simulink model "idblocks"  (Simulink 6.3)
settings: Solver=ode45  StartTime=0.0  StopTime=10.0  RelTol=1e-3
values from neighbouring files (symbols this model uses):
  f = fn(1)    [fgnewt.m]    (also in m_mvid.m = TR*f*inv(TR))
  N = ss(AN,BN,CN,DN)    [ncf.m]
  q = TR*q    [m_mvid.m]
  Q = Q0*It; end    [adils.m]    (also in cfesens.m = [q1 q6;q2 q4;q3 q5]; dia_con.m = diag(x(1:m)); dia_con1.m = diag(x(1:m)); dia_conl.m = eye(m,m))
undefined symbols (not defined in the file or in its folder): f_ord, lambda, npar, QKF, rho, Tsa, u_noise, y_noise
libraries: simulink x22
settings Model: LastModifiedBy=Kostas Tsakalis  StrictBusMsg=None
settings OptimizationCC: InlineInvariantSignals=on

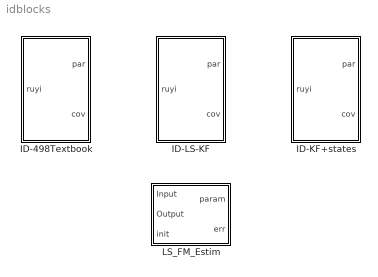
== system idblocks ==
  ID-498Textbook : Subsystem
  ID-KF+states : Subsystem
  ID-LS-KF : Subsystem
  LS_FM_Estim : Subsystem  mask{Tsa=0.01, N=4, thmin=-100, thmax=100, lambda=.9995, rho=1e5, y_noise=1e-6, u_noise=1e-6, Q=1e-8, lsgrad=1}
      mask prompts: Tsa "Tsample"; N "Order"; thmin "Min parameter"; thmax "Max Parameter"; rho "rho - Init cov"; y_noise "output regularization noise"; u_noise "input regularization noise"; Q "Q-dirft"; lsgrad "LS-gradient switch"

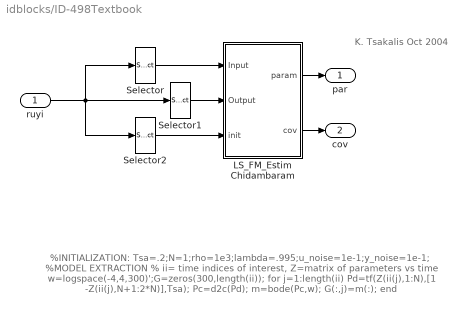
== system idblocks/ID-498Textbook ==
  note: %INITIALIZATION:
      | Tsa=.2;N=1;rho=1e3;lambda=.995;u_noise=1e-1;y_noise=1e-1;
      |
      | %MODEL EXTRACTION
      | % ii= time indices of interest, Z=matrix of parameters vs time
      | w=logspace(-4,4,300)';G=zeros(300,length(ii));
      | for j=1:length(ii)
      |    Pd=tf(Z(ii(j),1:N),[1 -Z(ii(j),N+1:2*N)],Tsa);
      |    Pc=d2c(Pd); m=bode(Pc,w); G(:,j)=m(:);
      | end
  note: K. Tsakalis
      | Oct 2004
  ruyi : Inport
  LS_FM_Estim Chidambaram : Subsystem
  Selector : Selector  Elements=2  InputPortWidth=4
  Selector1 : Selector  Elements=3  InputPortWidth=4
  Selector2 : Selector  Elements=4  InputPortWidth=4
  par : Outport
  cov : Outport  Port=2
  wires:
  Selector2/1 -> LS_FM_Estim Chidambaram/3(init)
  Selector1/1 -> LS_FM_Estim Chidambaram/2(Output)
  ruyi/1 -> Selector2/1, Selector1/1, Selector/1
  Selector/1 -> LS_FM_Estim Chidambaram/1(Input)
  LS_FM_Estim Chidambaram/1(param) -> par/1
  LS_FM_Estim Chidambaram/2(cov) -> cov/1

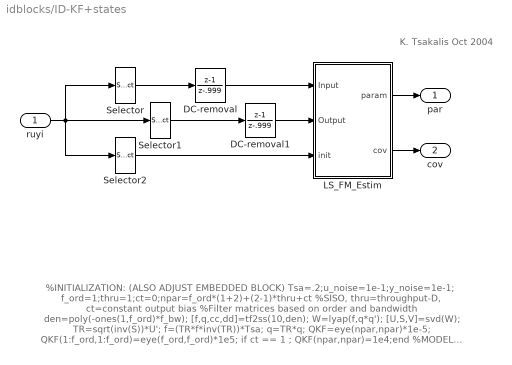
== system idblocks/ID-KF+states ==
  note: %INITIALIZATION: (ALSO ADJUST EMBEDDED BLOCK)
      | Tsa=.2;u_noise=1e-1;y_noise=1e-1;
      | f_ord=1;thru=1;ct=0;npar=f_ord*(1+2)+(2-1)*thru+ct
      | %SISO, thru=throughput-D, ct=constant output bias
      | %Filter matrices based on order and bandwidth
      | den=poly(-ones(1,f_ord)*f_bw); [f,q,cc,dd]=tf2ss(10,den);  W=lyap(f,q*q'); [U,S,V]=svd(W);
      | TR=sqrt(inv(S))*U';  f=(TR*f*inv(TR))*Tsa;  q=TR*q;
      | QKF=eye(npar,npar)*1e-5;   QKF(1:f_ord,1:f_ord)=eye(f_ord,f_ord)*1e5;
      | if ct == 1 ; QKF(npar,npar)=1e4;end
      |
      | %MODEL EXTRACTION
      | % ii= indices of points, Z=matrix of parameters vs time
      | w=logspace(-4,4,300)';G=zeros(300,length(ii));
      | for j=1:length(ii)
      |    q1=Z(ii(j),1:f_ord); q2=Z(ii(j),f_ord+1:2*f_ord); q3=Z(ii(j),mm-1*ct)*thru;
      |    Pd=ss(eye(size(f))+f'+q1'*q,q2'+q1'*q3,q,q3,Tsa); Pc=d2c(Pd); m=bode(Pc,w); G(:,j)=m(:);
      | end
  note: K. Tsakalis
      | Oct 2004
  ruyi : Inport
  DC-removal : DiscreteTransferFcn  Numerator=[1 -1]  Denominator=[1 -.999]  SampleTime=Tsa
  DC-removal1 : DiscreteTransferFcn  Numerator=[1 -1]  Denominator=[1 -.999]  SampleTime=Tsa
  LS_FM_Estim : Subsystem
  Selector : Selector  Elements=2  InputPortWidth=4
  Selector1 : Selector  Elements=3  InputPortWidth=4
  Selector2 : Selector  Elements=4  InputPortWidth=4
  par : Outport
  cov : Outport  Port=2
  wires:
  Selector2/1 -> LS_FM_Estim/3(init)
  Selector1/1 -> DC-removal1/1
  ruyi/1 -> Selector2/1, Selector1/1, Selector/1
  Selector/1 -> DC-removal/1
  LS_FM_Estim/1(param) -> par/1
  LS_FM_Estim/2(cov) -> cov/1
  DC-removal/1 -> LS_FM_Estim/1(Input)
  DC-removal1/1 -> LS_FM_Estim/2(Output)

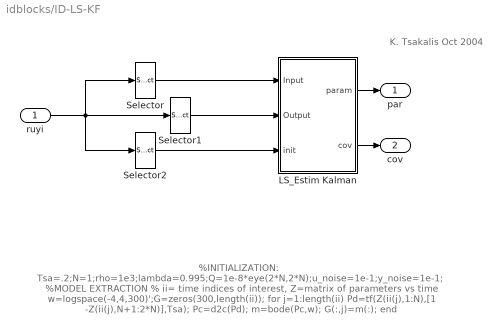
== system idblocks/ID-LS-KF ==
  note: %INITIALIZATION:
      | Tsa=.2;N=1;rho=1e3;lambda=0.995;Q=1e-8*eye(2*N,2*N);u_noise=1e-1;y_noise=1e-1;
      |
      | %MODEL EXTRACTION
      | % ii= time indices of interest, Z=matrix of parameters vs time
      | w=logspace(-4,4,300)';G=zeros(300,length(ii));
      | for j=1:length(ii)
      |    Pd=tf(Z(ii(j),1:N),[1 -Z(ii(j),N+1:2*N)],Tsa);
      |    Pc=d2c(Pd); m=bode(Pc,w); G(:,j)=m(:);
      | end
  note: K. Tsakalis
      | Oct 2004
  ruyi : Inport
  LS_Estim Kalman : Subsystem
  Selector : Selector  Elements=2  InputPortWidth=4
  Selector1 : Selector  Elements=3  InputPortWidth=4
  Selector2 : Selector  Elements=4  InputPortWidth=4
  par : Outport
  cov : Outport  Port=2
  wires:
  LS_Estim Kalman/2(cov) -> cov/1
  LS_Estim Kalman/1(param) -> par/1
  Selector/1 -> LS_Estim Kalman/1(Input)
  ruyi/1 -> Selector/1, Selector1/1, Selector2/1
  Selector1/1 -> LS_Estim Kalman/2(Output)
  Selector2/1 -> LS_Estim Kalman/3(init)

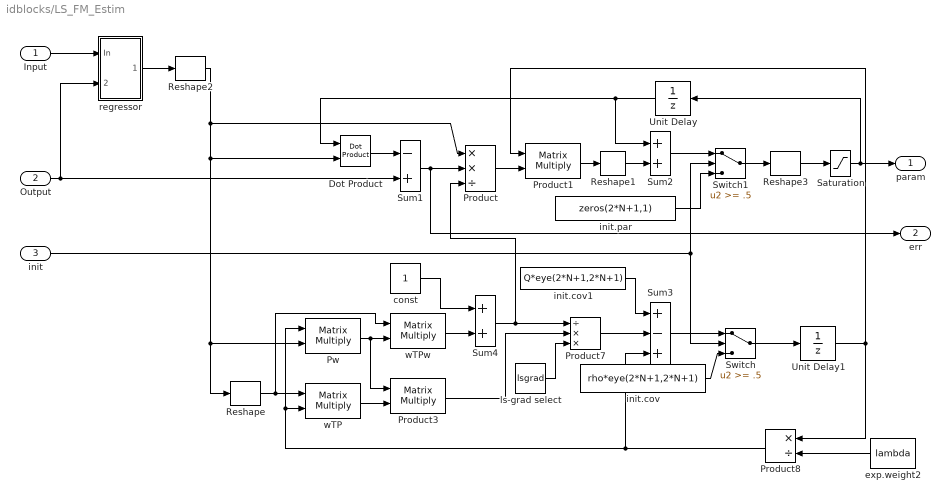
== system idblocks/LS_FM_Estim ==
  Input : Inport
  Output : Inport  Port=2
  init : Inport  Port=3
  Dot Product : simulink/Math Operations/Dot Product  InputSameDT=on  OutDataType=sfix(16)  OutScaling=2^-10  DoSatur=off
  Product : Product  Inputs=**/  RndMeth=Zero
  Product1 : Product  Multiplication=Matrix(*)  RndMeth=Zero
  Product3 : Product  Multiplication=Matrix(*)  RndMeth=Zero
  Product7 : Product  Inputs=/**  RndMeth=Zero
  Product8 : Product  Orientation=left  Inputs=*/  RndMeth=Zero
  Pw : Product  Multiplication=Matrix(*)  RndMeth=Zero
  Reshape : simulink/Math Operations/Reshape  OutputDimensionality=Row vector  OutputDimensions=[1,1]
  Reshape1 : simulink/Math Operations/Reshape  OutputDimensionality=Column vector  OutputDimensions=[1,1]
  Reshape2 : simulink/Math Operations/Reshape  OutputDimensionality=Column vector  OutputDimensions=[1,1]
  Reshape3 : simulink/Math Operations/Reshape  OutputDimensionality=1-D array  OutputDimensions=[1,1]
  Saturation : Saturate  UpperLimit=thmax  LowerLimit=thmin
  Sum1 : Sum  Inputs=-+  SaturateOnIntegerOverflow=on
  Sum2 : Sum  Inputs=2  SaturateOnIntegerOverflow=on
  Sum3 : Sum  Inputs=+-+  SaturateOnIntegerOverflow=on
  Sum4 : Sum  Inputs=2  SaturateOnIntegerOverflow=on
  Switch : Switch  Threshold=.5
  Switch1 : Switch  Threshold=.5
  Unit Delay : UnitDelay  Orientation=left  SampleTime=Tsa
  Unit Delay1 : UnitDelay  X0=rho*eye(2*N+1,2*N+1)  SampleTime=Tsa
  const : Constant
  exp.weight2 : Constant  Orientation=left  Value=lambda
  init.cov : Constant  Value=rho*eye(2*N+1,2*N+1)  VectorParams1D=off
  init.cov1 : Constant  Value=Q*eye(2*N+1,2*N+1)  VectorParams1D=off  SampleTime=Tsa
  init.par : Constant  Value=zeros(2*N+1,1)  VectorParams1D=off  SampleTime=Tsa
  ls-grad select : Constant  Value=lsgrad
  regressor : Subsystem
  wTP : Product  Multiplication=Matrix(*)  RndMeth=Zero
  wTPw : Product  Multiplication=Matrix(*)  RndMeth=Zero
  param : Outport
  err : Outport  Port=2
  wires:
  Saturation/1 -> Unit Delay/1, param/1
  Switch1/1 -> Reshape3/1
  init.cov1/1 -> Sum3/1
  Product7/1 -> Sum3/2
  exp.weight2/1 -> Product8/2
  Product8/1 -> Sum3/3, wTP/2, Pw/1
  ls-grad select/1 -> Product7/3
  Sum3/1 -> Switch/1
  const/1 -> Sum4/1
  regressor/1(regr) -> Reshape2/1
  Input/1 -> regressor/1(In)
  Reshape3/1 -> Saturation/1
  Reshape1/1 -> Sum2/2
  Dot Product/1 -> Sum1/1
  Output/1 -> regressor/2(out), Sum1/2
  Sum1/1 -> err/1, Product/2
  Product/1 -> Product1/2
  Reshape2/1 -> Dot Product/2, Reshape/1, Pw/2, Product/1
  Reshape/1 -> wTP/1, wTPw/1
  Product1/1 -> Reshape1/1
  wTP/1 -> Product3/2
  Product3/1 -> Product7/2
  Pw/1 -> Product3/1, wTPw/2
  wTPw/1 -> Sum4/2
  Sum4/1 -> Product/3, Product7/1
  Unit Delay1/1 -> Product8/1, Product1/1
  init.cov/1 -> Switch/3
  init/1 -> Switch/2, Switch1/2
  Switch/1 -> Unit Delay1/1
  Sum2/1 -> Switch1/1
  init.par/1 -> Switch1/3
  Unit Delay/1 -> Dot Product/1, Sum2/1

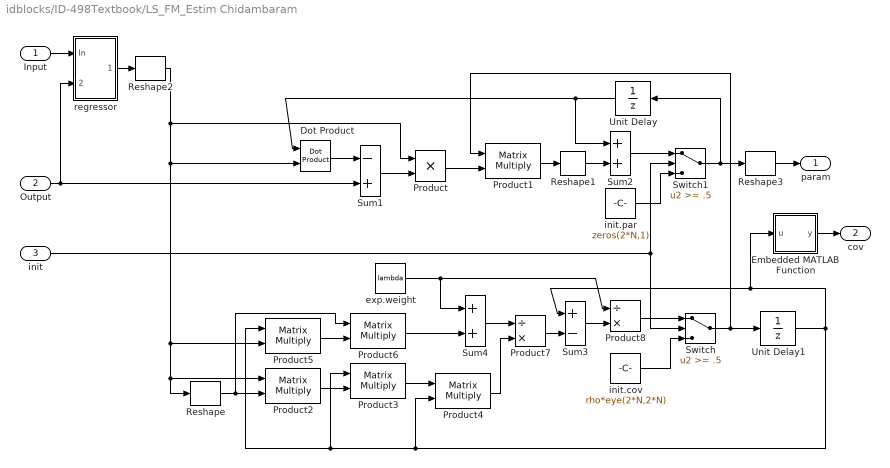
== system idblocks/ID-498Textbook/LS_FM_Estim Chidambaram ==
  Input : Inport
  Output : Inport  Port=2
  init : Inport  Port=3
  Dot Product : simulink/Math Operations/Dot Product  InputSameDT=on  OutDataType=sfix(16)  OutScaling=2^-10  DoSatur=off
  Embedded MATLAB Function : Stateflow chart
  Product : Product  RndMeth=Zero
  Product{1..6} (6 alike) : Product  Multiplication=Matrix(*)  RndMeth=Zero
  Product7 : Product  Inputs=/*  RndMeth=Zero
  Product8 : Product  Inputs=/*  RndMeth=Zero
  Reshape : simulink/Math Operations/Reshape  OutputDimensionality=Row vector  OutputDimensions=[1,1]
  Reshape1 : simulink/Math Operations/Reshape  OutputDimensionality=Column vector  OutputDimensions=[1,1]
  Reshape2 : simulink/Math Operations/Reshape  OutputDimensionality=Column vector  OutputDimensions=[1,1]
  Reshape3 : simulink/Math Operations/Reshape  OutputDimensionality=1-D array  OutputDimensions=[1,1]
  Sum1 : Sum  Inputs=-+  SaturateOnIntegerOverflow=on
  Sum2 : Sum  Inputs=2  SaturateOnIntegerOverflow=on
  Sum3 : Sum  Inputs=+-  SaturateOnIntegerOverflow=on
  Sum4 : Sum  Inputs=2  SaturateOnIntegerOverflow=on
  Switch : Switch  Threshold=.5
  Switch1 : Switch  Threshold=.5
  Unit Delay : UnitDelay  Orientation=left  SampleTime=Tsa
  Unit Delay1 : UnitDelay  SampleTime=Tsa
  exp.weight : Constant  Value=lambda  SampleTime=Tsa
  init.cov : Constant  Value=rho*eye(2*N,2*N)  VectorParams1D=off  SampleTime=Tsa
  init.par : Constant  Value=zeros(2*N,1)  VectorParams1D=off  SampleTime=Tsa
  regressor : Subsystem
  param : Outport
  cov : Outport  Port=2
  wires:
  Embedded MATLAB Function/1(y) -> cov/1
  regressor/1(regr) -> Reshape2/1
  Input/1 -> regressor/1(In)
  Reshape3/1 -> param/1
  Reshape1/1 -> Sum2/2
  Dot Product/1 -> Sum1/1
  Output/1 -> regressor/2(out), Sum1/2
  Sum1/1 -> Product/2
  Product/1 -> Product1/2
  Reshape2/1 -> Dot Product/2, Product5/2, Product2/1, Reshape/1, Product/1
  Reshape/1 -> Product6/1, Product2/2
  Product1/1 -> Reshape1/1
  Product2/1 -> Product3/2
  Product3/1 -> Product4/1
  Product5/1 -> Product6/2
  Product6/1 -> Sum4/2
  Product4/1 -> Product7/2
  Sum4/1 -> Product7/1
  Product7/1 -> Sum3/2
  Unit Delay1/1 -> Embedded MATLAB Function/1(u), Sum3/1, Product5/1, Product3/1, Product4/2
  Sum3/1 -> Product8/2
  exp.weight/1 -> Sum4/1, Product8/1
  Product8/1 -> Switch/1
  init.cov/1 -> Switch/3
  init/1 -> Switch/2, Switch1/2
  Switch/1 -> Product1/1, Unit Delay1/1
  Sum2/1 -> Switch1/1
  init.par/1 -> Switch1/3
  Unit Delay/1 -> Dot Product/1, Sum2/1
  Switch1/1 -> Reshape3/1, Unit Delay/1

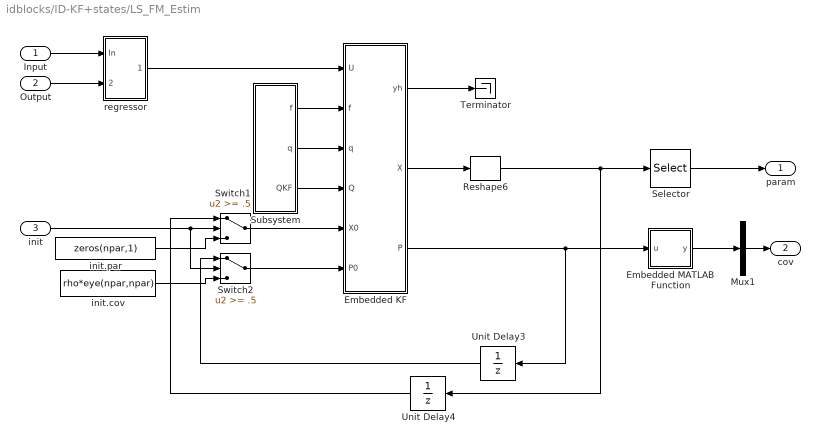
== system idblocks/ID-KF+states/LS_FM_Estim ==
  Input : Inport
  Output : Inport  Port=2
  init : Inport  Port=3
  Embedded KF : Stateflow chart
  Embedded MATLAB Function : Stateflow chart
  Mux1 : Mux  Inputs=1
  Reshape6 : simulink/Math Operations/Reshape  OutputDimensionality=1-D array  OutputDimensions=[npar,npar]
  Selector : Selector  Elements=[f_ord+1:npar]  InputPortWidth=npar
  Subsystem : Subsystem
  Switch1 : Switch  Threshold=.5
  Switch2 : Switch  Threshold=.5
  Terminator : Terminator
  Unit Delay3 : UnitDelay  Orientation=left  SampleTime=Tsa
  Unit Delay4 : UnitDelay  Orientation=left  SampleTime=Tsa
  init.cov : Constant  Value=rho*eye(npar,npar)  VectorParams1D=off  SampleTime=Tsa
  init.par : Constant  Value=zeros(npar,1)  VectorParams1D=off  SampleTime=Tsa
  regressor : Subsystem
  param : Outport
  cov : Outport  Port=2
  wires:
  Selector/1 -> param/1
  Embedded KF/3(P) -> Unit Delay3/1, Embedded MATLAB Function/1(u)
  Embedded KF/2(X) -> Reshape6/1
  Unit Delay3/1 -> Switch2/1
  init.cov/1 -> Switch2/3
  Switch2/1 -> Embedded KF/6(P0)
  Unit Delay4/1 -> Switch1/1
  Switch1/1 -> Embedded KF/5(X0)
  init.par/1 -> Switch1/3
  init/1 -> Switch2/2, Switch1/2
  Subsystem/2(q) -> Embedded KF/3(q)
  Subsystem/1(f) -> Embedded KF/2(f)
  Reshape6/1 -> Unit Delay4/1, Selector/1
  Mux1/1 -> cov/1
  Embedded MATLAB Function/1(y) -> Mux1/1
  regressor/1(regr) -> Embedded KF/1(U)
  Input/1 -> regressor/1(In)
  Output/1 -> regressor/2(out)
  Embedded KF/1(yh) -> Terminator/1
  Subsystem/3(QKF) -> Embedded KF/4(Q)

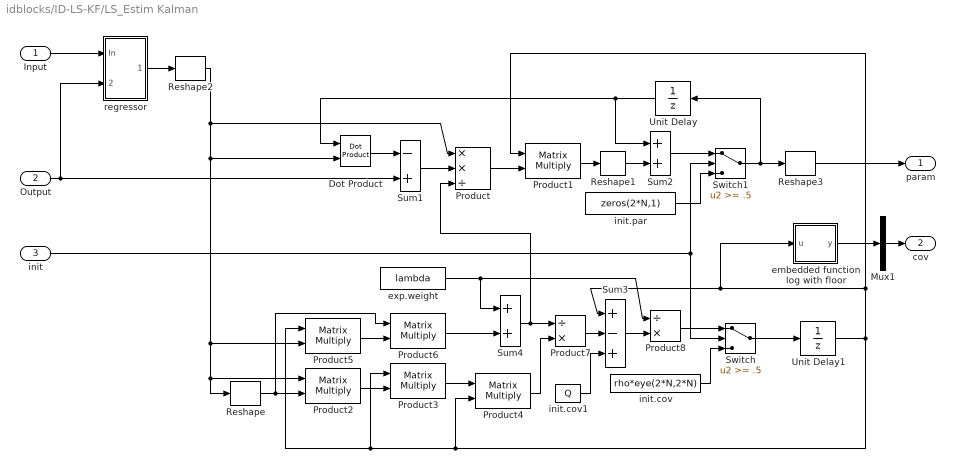
== system idblocks/ID-LS-KF/LS_Estim Kalman ==
  Input : Inport
  Output : Inport  Port=2
  init : Inport  Port=3
  Dot Product : simulink/Math Operations/Dot Product  InputSameDT=on  OutDataType=sfix(16)  OutScaling=2^-10  DoSatur=off
  Mux1 : Mux  Inputs=1
  Product : Product  Inputs=**/  RndMeth=Zero
  Product{1..6} (6 alike) : Product  Multiplication=Matrix(*)  RndMeth=Zero
  Product7 : Product  Inputs=/*  RndMeth=Zero
  Product8 : Product  Inputs=/*  RndMeth=Zero
  Reshape : simulink/Math Operations/Reshape  OutputDimensionality=Row vector  OutputDimensions=[1,1]
  Reshape1 : simulink/Math Operations/Reshape  OutputDimensionality=Column vector  OutputDimensions=[1,1]
  Reshape2 : simulink/Math Operations/Reshape  OutputDimensionality=Column vector  OutputDimensions=[1,1]
  Reshape3 : simulink/Math Operations/Reshape  OutputDimensionality=1-D array  OutputDimensions=[1,1]
  Sum1 : Sum  Inputs=-+  SaturateOnIntegerOverflow=on
  Sum2 : Sum  Inputs=2  SaturateOnIntegerOverflow=on
  Sum3 : Sum  Inputs=+-+  SaturateOnIntegerOverflow=on
  Sum4 : Sum  Inputs=2  SaturateOnIntegerOverflow=on
  Switch : Switch  Threshold=.5
  Switch1 : Switch  Threshold=.5
  Unit Delay : UnitDelay  Orientation=left  SampleTime=Tsa
  Unit Delay1 : UnitDelay  X0=rho*eye(2*N,2*N)  SampleTime=Tsa
  embedded function log with floor : Stateflow chart
  exp.weight : Constant  Value=lambda  SampleTime=Tsa
  init.cov : Constant  Value=rho*eye(2*N,2*N)  VectorParams1D=off  SampleTime=Tsa
  init.cov1 : Constant  Value=Q  VectorParams1D=off  SampleTime=Tsa
  init.par : Constant  Value=zeros(2*N,1)  VectorParams1D=off  SampleTime=Tsa
  regressor : Subsystem
  param : Outport
  cov : Outport  Port=2
  wires:
  Switch1/1 -> Unit Delay/1, Reshape3/1
  Unit Delay/1 -> Sum2/1, Dot Product/1
  init.par/1 -> Switch1/3
  Sum2/1 -> Switch1/1
  Switch/1 -> Unit Delay1/1
  init/1 -> Switch1/2, Switch/2
  init.cov/1 -> Switch/3
  Product8/1 -> Switch/1
  exp.weight/1 -> Product8/1, Sum4/1
  Sum3/1 -> Product8/2
  Unit Delay1/1 -> Product4/2, Product3/1, Product5/1, Sum3/1, embedded function log with floor/1(u), Product1/1
  Product7/1 -> Sum3/2
  Sum4/1 -> Product7/1, Product/3
  Product4/1 -> Product7/2
  Product6/1 -> Sum4/2
  Product5/1 -> Product6/2
  Product3/1 -> Product4/1
  Product2/1 -> Product3/2
  Product1/1 -> Reshape1/1
  Reshape/1 -> Product2/2, Product6/1
  Reshape2/1 -> Product/1, Reshape/1, Product2/1, Product5/2, Dot Product/2
  Product/1 -> Product1/2
  Sum1/1 -> Product/2
  Output/1 -> regressor/2(out), Sum1/2
  Dot Product/1 -> Sum1/1
  Reshape1/1 -> Sum2/2
  Reshape3/1 -> param/1
  Input/1 -> regressor/1(In)
  regressor/1(regr) -> Reshape2/1
  embedded function log with floor/1(y) -> Mux1/1
  Mux1/1 -> cov/1
  init.cov1/1 -> Sum3/3

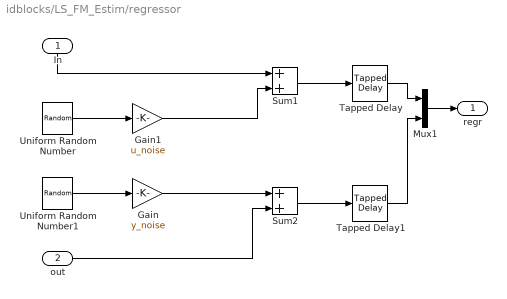
== system idblocks/LS_FM_Estim/regressor ==
  In : Inport  Orientation=down
  out : Inport  Port=2
  Gain : Gain  Gain=y_noise
  Gain1 : Gain  Gain=u_noise
  Mux1 : Mux  Inputs=2
  Sum1 : Sum  SaturateOnIntegerOverflow=on
  Sum2 : Sum  SaturateOnIntegerOverflow=on
  Tapped Delay : simulink/Discrete/Tapped Delay  vinit=0  samptime=Tsa  NumDelays=N  DelayOrder=Newest  includeCurrent=on
  Tapped Delay1 : simulink/Discrete/Tapped Delay  vinit=0  samptime=Tsa  NumDelays=N  DelayOrder=Newest  includeCurrent=off
  Uniform Random Number : UniformRandomNumber  SampleTime=Tsa
  Uniform Random Number1 : UniformRandomNumber  Seed=1  SampleTime=Tsa
  regr : Outport
  wires:
  Tapped Delay1/1 -> Mux1/2
  Tapped Delay/1 -> Mux1/1
  Mux1/1 -> regr/1
  Sum1/1 -> Tapped Delay/1
  In/1 -> Sum1/1
  Uniform Random Number/1 -> Gain1/1
  Sum2/1 -> Tapped Delay1/1
  Uniform Random Number1/1 -> Gain/1
  out/1 -> Sum2/2
  Gain/1 -> Sum2/1
  Gain1/1 -> Sum1/2

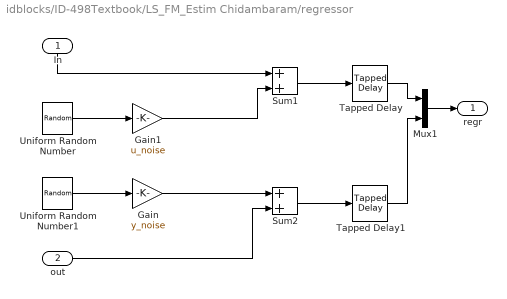
== system idblocks/ID-498Textbook/LS_FM_Estim Chidambaram/regressor ==
  In : Inport  Orientation=down
  out : Inport  Port=2
  Gain : Gain  Gain=y_noise
  Gain1 : Gain  Gain=u_noise
  Mux1 : Mux  Inputs=2
  Sum1 : Sum  SaturateOnIntegerOverflow=on
  Sum2 : Sum  SaturateOnIntegerOverflow=on
  Tapped Delay : simulink/Discrete/Tapped Delay  vinit=0  samptime=Tsa  NumDelays=N  DelayOrder=Oldest  includeCurrent=off
  Tapped Delay1 : simulink/Discrete/Tapped Delay  vinit=0  samptime=Tsa  NumDelays=N  DelayOrder=Oldest  includeCurrent=off
  Uniform Random Number : UniformRandomNumber  SampleTime=Tsa
  Uniform Random Number1 : UniformRandomNumber  Seed=1  SampleTime=Tsa
  regr : Outport
  wires:
  Tapped Delay1/1 -> Mux1/2
  Tapped Delay/1 -> Mux1/1
  Mux1/1 -> regr/1
  Sum1/1 -> Tapped Delay/1
  In/1 -> Sum1/1
  Uniform Random Number/1 -> Gain1/1
  Sum2/1 -> Tapped Delay1/1
  Uniform Random Number1/1 -> Gain/1
  out/1 -> Sum2/2
  Gain/1 -> Sum2/1
  Gain1/1 -> Sum1/2

== system idblocks/ID-KF+states/LS_FM_Estim/Subsystem ==
  init.Q : Constant  Value=QKF  SampleTime=Tsa
  init.cov1 : Constant  Value=f  SampleTime=Tsa
  init.cov2 : Constant  Value=q  SampleTime=Tsa
  f : Outport
  q : Outport  Port=2
  QKF : Outport  Port=3
  wires:
  init.cov2/1 -> q/1
  init.cov1/1 -> f/1
  init.Q/1 -> QKF/1

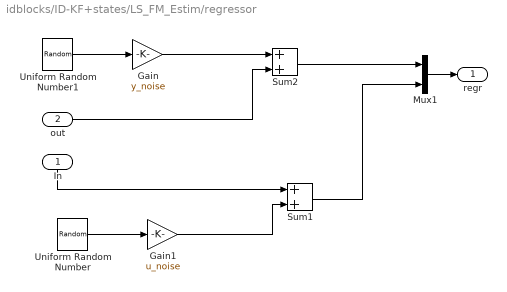
== system idblocks/ID-KF+states/LS_FM_Estim/regressor ==
  In : Inport  Orientation=down
  out : Inport  Port=2
  Gain : Gain  Gain=y_noise
  Gain1 : Gain  Gain=u_noise
  Mux1 : Mux  Inputs=2
  Sum1 : Sum  SaturateOnIntegerOverflow=on
  Sum2 : Sum  SaturateOnIntegerOverflow=on
  Uniform Random Number : UniformRandomNumber  SampleTime=Tsa
  Uniform Random Number1 : UniformRandomNumber  Seed=1  SampleTime=Tsa
  regr : Outport
  wires:
  Sum1/1 -> Mux1/2
  Sum2/1 -> Mux1/1
  Mux1/1 -> regr/1
  In/1 -> Sum1/1
  Uniform Random Number/1 -> Gain1/1
  Uniform Random Number1/1 -> Gain/1
  out/1 -> Sum2/2
  Gain/1 -> Sum2/1
  Gain1/1 -> Sum1/2

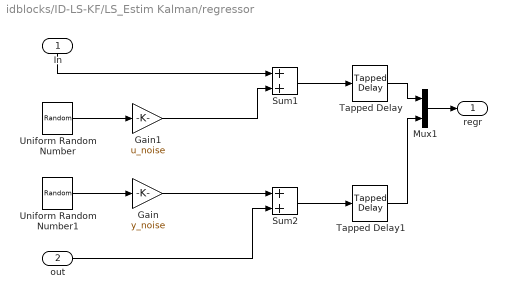
== system idblocks/ID-LS-KF/LS_Estim Kalman/regressor ==
  In : Inport  Orientation=down
  out : Inport  Port=2
  Gain : Gain  Gain=y_noise
  Gain1 : Gain  Gain=u_noise
  Mux1 : Mux  Inputs=2
  Sum1 : Sum  SaturateOnIntegerOverflow=on
  Sum2 : Sum  SaturateOnIntegerOverflow=on
  Tapped Delay : simulink/Discrete/Tapped Delay  vinit=0  samptime=Tsa  NumDelays=N  DelayOrder=Oldest  includeCurrent=off
  Tapped Delay1 : simulink/Discrete/Tapped Delay  vinit=0  samptime=Tsa  NumDelays=N  DelayOrder=Oldest  includeCurrent=off
  Uniform Random Number : UniformRandomNumber  SampleTime=Tsa
  Uniform Random Number1 : UniformRandomNumber  Seed=1  SampleTime=Tsa
  regr : Outport
  wires:
  Gain1/1 -> Sum1/2
  Gain/1 -> Sum2/1
  out/1 -> Sum2/2
  Uniform Random Number1/1 -> Gain/1
  Sum2/1 -> Tapped Delay1/1
  Uniform Random Number/1 -> Gain1/1
  In/1 -> Sum1/1
  Sum1/1 -> Tapped Delay/1
  Mux1/1 -> regr/1
  Tapped Delay/1 -> Mux1/1
  Tapped Delay1/1 -> Mux1/2

== matlab function ID-KF+states/LS_FM_Estim/Embedded KF ==
  data: yh output inherited; U input inherited; X output double; f input inherited; q input inherited; Q input inherited; X0 input inherited; P0 input inherited; P output inherited
function [yh,X,P] = fcn(U,f,q,Q,X0,P0)
% nin = # out + in
%
nin=2;
f_ord=1; thru=1; ct=0;
npar=f_ord*(1+nin)+(nin-1)*thru+ct;
y=U(1); u=U(2);

A=zeros(npar,npar);       C=zeros(1,npar);         C(1:f_ord)=q';
Xhi=1e9*ones(npar,1);    Xlo=-1e9*ones(npar,1);

A(1:f_ord,1:f_ord)=f';
A(1:f_ord,f_ord+1:2*f_ord)=diag(ones(f_ord,1))*y;
ii=1;
A(1:f_ord,(ii+1)*f_ord+1:(ii+2)*f_ord)=diag(ones(f_ord,1))*u(ii);
if thru==1
    if ct==1, C(npar-nin+1:npar)=[u',1];  else,  C(npar-nin+2:npar)=u';  end
else
    if ct==1, C(npar:npar)=1;   end
end
AD=eye(size(A))+A;
P=AD*P0*AD'+Q-AD*P0*C'*C*P0*AD'/(C*P0*C'+1);
L=-AD*P0*C'/(C*P0*C'+1);   yh=C*X0;
X=AD*X0+L*(yh-y);    
%X=sat(X,Xhi,Xlo);

== matlab function ID-498Textbook/LS_FM_Estim Chidambaram/Embedded MATLAB Function ==
  data: u input inherited; y output double
function y = fcn(u)
% This block supports an embeddable subset of the MATLAB language.
% See the help menu for details. 

y = (svd(u));
y = log(max(1e-6,y))/log(10);

== matlab function ID-LS-KF/LS_Estim Kalman/embedded function log with floor ==
  data: u input inherited; y output double
function y = fcn(u)
% This block supports an embeddable subset of the MATLAB language.
% See the help menu for details. 

y = (svd(u));
y = log(max(1e-9,y))/log(10);

== matlab function ID-KF+states/LS_FM_Estim/Embedded MATLAB Function ==
  data: u input inherited; y output double
function y = fcn(u)
% This block supports an embeddable subset of the MATLAB language.
% See the help menu for details. 

y = (svd(u));
y = log(max(1e-9,y))/log(10);
